simulink model "Model_PID"  (R2020b)
settings: Solver=ode4  StartTime=0.0  StopTime=1000  FixedStep=0.01  RelTol=1e-3
undefined symbols (not defined in the file): B, D, E_c, gama_c, gama_vjet, H, Iz, Kdpsi, Kdx, Kipsi, Kix, Kppsi, Kpx, Kurs_poc, L, m, N_c, Nr, Nrdot, Nrr, Nv, Polozaj_poc_E, Polozaj_poc_N, r_o, ro, ro_vj, T, V_c, V_vj, Xu, Xudot, Yr, Yrdot, Yv, Yvdot
libraries: simulink_extras x8, simulink x2
settings Model: Creator=Luka  LastModifiedBy=Luka
settings SolverCC: AlgebraicLoopSolver=LineSearch

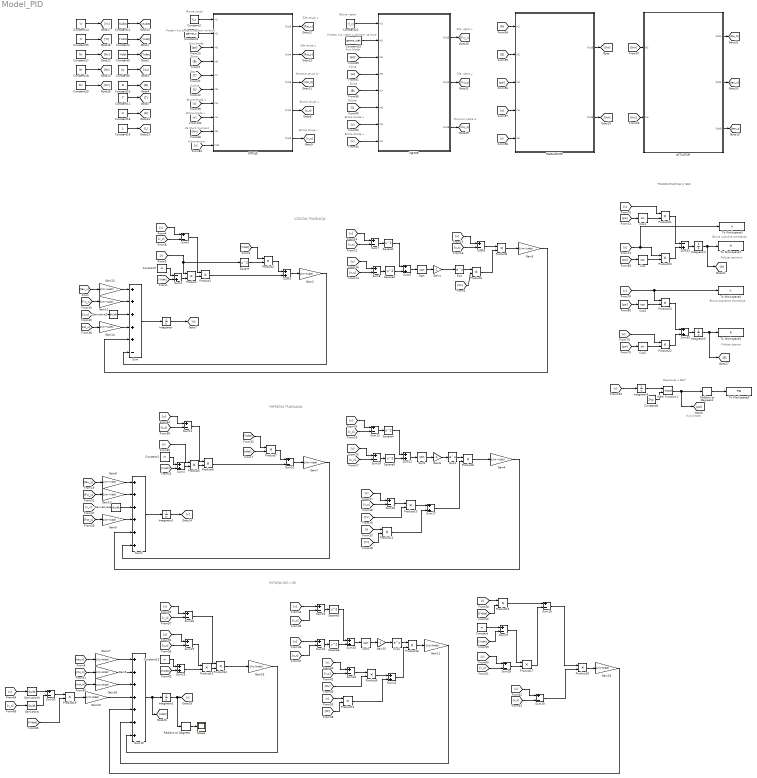
== system Model_PID ==
  note: Brzina struje v
  note: Brzina struje u
  note: Kutna brzina
  note: UZDUŽNA TRANSLACIJA
  note: POPREČNA TRANSLACIJA
  note: ROTACIJA OKO z OSI
  note: TRANSFORAMCIJA U NED
  note: Položaj istočno
  note: Položaj sjeverno
  note: Brzina uzdužna translacija
  note: Brzina poprečna translacija
  note: Visina
  note: Sila vjetra x
  note: Brzina vjetra
  note: Sila vjetra y
  note: Moment vjetra N
  note: Duljina
  note: Širina
  note: Pocetni kut vjetra s obzirom na brod
  note: Kurs broda
  note: Brzina broda u
  note: Brzina broda v
  note: Sila struje y
  note: Gaz
  note: Brzina struje
  note: Pocetni kut struje s obzirom na brod
  note: Sila struje x
  note: Duljina
  note: Kurs broda
  note: Moment struje N
  note: Širina
  note: Za Munk moment
  note: Brzina broda v
  note: Brzina broda u
  note: Mapiranje u 360°
  note: Kurs broda
  AKTUATOR : Subsystem
  Constant{,1,7,13} (4 alike) : Constant  Value=m
  Constant10 : Constant  Value=B
  Constant11 : Constant  Value=T
  Constant12 : Constant  Value=Xudot
  Constant14 : Constant  Value=Yv
  Constant15 : Constant  Value=Yr
  Constant16 : Constant  Value=H
  Constant17 : Constant  Value=Nv
  Constant18 : Constant  Value=Nr
  Constant19 : Constant  Value=L
  Constant2 : Constant  Value=V_c
  Constant20 : Constant  Value=Nrr
  Constant24 : Constant  Value=V_vj
  Constant25 : Constant  Value=gama_vjet
  Constant3 : Constant  Value=gama_c
  Constant4 : Constant  Value=Yvdot
  Constant5 : Constant  Value=Yrdot
  Constant6 : Constant  Value=Xu
  Constant8 : Constant  Value=2*pi
  Cos : Trigonometry  Operator=cos
  Cos1 : Trigonometry
  Cos2 : Trigonometry
  Cos3 : Trigonometry  Operator=cos
  Derivative{,1..3} (4 alike) : Derivative
  Exp : Math  SaturateOnIntegerOverflow=on
  Exp1 : Math  SaturateOnIntegerOverflow=on
  Exp2 : Math  SaturateOnIntegerOverflow=on
  Gain1 : Gain  Gain=-1
  Gain{4,7..10} (5 alike) : Gain  Gain=1/(m-Yvdot)
  Gain{5,11,16..20} (7 alike) : Gain  Gain=1/(Iz-Nrdot)
  Gain{2..3,12..14} (5 alike) : Gain  Gain=1/(m-Xudot)
  Gain15 : Gain  Gain=-1
  Gain6 : Gain  Gain=-1
  Integrator : Integrator
  Integrator1 : Integrator
  Integrator2 : Integrator
  Integrator4 : Integrator  InitialCondition=Polozaj_poc_N
  Integrator5 : Integrator  InitialCondition=Polozaj_poc_E
  Integrator6 : Integrator  InitialCondition=Kurs_poc
  Math Function1 : Math  Operator=mod  SaturateOnIntegerOverflow=on
  Product{,1..23} (24 alike) : Product
  REGULATOR : Subsystem
  Radians to Degrees : simulink_extras/Transformations/Radians to Degrees
  Radians to Degrees1 : simulink_extras/Transformations/Radians to Degrees
  STRUJE : Subsystem
  Scope : Scope
  Sqrt : Sqrt  SaturateOnIntegerOverflow=on
  Sqrt1 : Sqrt  SaturateOnIntegerOverflow=on
  Sqrt2 : Sqrt  SaturateOnIntegerOverflow=on
  Square{,1..6} (7 alike) : Math  Operator=square  SaturateOnIntegerOverflow=on
  Sum : Sum  Inputs=+++++-
  Sum1 : Sum  Inputs=++++++
  Sum{5,7..11,13..14,16,18..19,21..23,26..30} (19 alike) : Sum  Inputs=+-
  Sum{3..4,6,12,17,20,24..25,35} (9 alike) : Sum
  Sum15 : Sum  Inputs=+++++++
  Sum2 : Sum  Inputs=-+
  Sum32 : Sum  Inputs=-+
  To Workspace1 : ToWorkspace  VariableName=N  SaveFormat=Timeseries  SampleTime=-1
  To Workspace2 : ToWorkspace  VariableName=E  SaveFormat=Timeseries  SampleTime=-1
  To Workspace3 : ToWorkspace  VariableName=U  SaveFormat=Timeseries  SampleTime=-1
  To Workspace4 : ToWorkspace  VariableName=V  SaveFormat=Timeseries  SampleTime=-1
  To Workspace5 : ToWorkspace  VariableName=PSI  SaveFormat=Timeseries  SampleTime=-1
  VJETAR : Subsystem
  wires:
  Sum/1 -> Integrator/1
  Constant4/1 -> [Yvdot]
  Constant5/1 -> [Yrdot]
  Constant6/1 -> [Xu]
  Constant7/1 -> Sum2/1
  Sum2/1 -> Product/2
  [r] -> Square/1, Product/1
  [Yvdot] -> Sum2/2
  Constant10/1 -> [B]
  Constant11/1 -> [T]
  Product/1 -> Product1/2
  Product1/1 -> Sum3/2
  Square/1 -> Product2/2
  [Yrdot] -> Product2/1
  Product2/1 -> Sum3/1
  [v] -> Sum5/1
  [v_c] -> Sum5/2
  Sum5/1 -> Product1/1
  [v] -> Sum7/1
  [v_c] -> Sum7/2
  Sum7/1 -> Square1/1
  [u_c] -> Sum8/2
  [u] -> Sum8/1
  Sum8/1 -> Square2/1
  Square2/1 -> Sum6/2
  Square1/1 -> Sum6/1
  Sum6/1 -> Sqrt/1
  Exp/1 -> Product3/1
  [Xu] -> Product3/2
  [u_c] -> Sum9/2
  [u] -> Sum9/1
  Product3/1 -> Product4/2
  Gain2/1 -> Sum/6
  Derivative1/1 -> Sum1/3
  [Fst_y] -> Gain9/1
  Gain7/1 -> Sum1/6
  Gain6/1 -> Exp1/1
  Sqrt1/1 -> Gain6/1
  [u] -> Sum11/1
  Product6/1 -> Sum10/2
  [v] -> Sum13/1
  Gain10/1 -> Sum1/2
  [u_c] -> Sum11/2
  Square5/1 -> Sum12/2
  Sum10/1 -> Gain7/1
  Product5/1 -> Product6/2
  [v_c] -> Derivative1/1
  [u_c] -> Sum14/2
  Sum13/1 -> Square4/1
  [u] -> Sum14/1
  Exp1/1 -> Product8/1
  [r] -> Product5/1
  Sum12/1 -> Sqrt1/1
  Sum14/1 -> Square5/1
  [Yrdot] -> Product7/1
  Sum1/1 -> Integrator1/1
  [v_c] -> Sum13/2
  [Fvj_y] -> Gain10/1
  Sum11/1 -> Product6/1
  Product7/1 -> Sum10/1
  Gain8/1 -> Sum1/1
  Integrator1/1 -> [v]
  Square4/1 -> Sum12/1
  [Xudot] -> Sum4/2
  Constant1/1 -> Sum4/1
  Sum4/1 -> Product5/2
  Product8/1 -> Gain4/1
  Product4/1 -> Gain3/1
  Derivative2/1 -> Sum/3
  [Fst_x] -> Gain14/1
  Gain12/1 -> Sum/2
  [Fvj_x] -> Gain12/1
  [tau_x] -> Gain13/1
  [u_c] -> Derivative2/1
  Sum3/1 -> Gain2/1
  Constant12/1 -> [Xudot]
  [rdot] -> Product7/2
  [v] -> Sum16/1
  [v_c] -> Sum16/2
  [Yv] -> Product10/2
  Product10/1 -> Sum17/1
  [r] -> Product11/1
  [Yr] -> Product11/2
  Product11/1 -> Sum17/2
  Sum17/1 -> Product8/2
  Constant14/1 -> [Yv]
  Constant15/1 -> [Yr]
  [v_c] -> Sum23/2
  Gain16/1 -> Sum15/7
  Gain18/1 -> Sum15/3
  [Mvj_N] -> Gain5/1
  Product14/1 -> Gain16/1
  Gain11/1 -> Sum15/6
  Product16/1 -> Gain11/1
  Gain15/1 -> Exp2/1
  Product12/1 -> Sum24/2
  [u] -> Sum19/1
  Sqrt2/1 -> Gain15/1
  Sum24/1 -> Product16/2
  [r] -> Product12/1
  Square6/1 -> Sum20/2
  [u_c] -> Sum19/2
  Gain5/1 -> Sum15/2
  [Nr] -> Product12/2
  Sum25/1 -> Product13/2
  [Xudot] -> Sum25/2
  Constant13/1 -> Sum25/1
  Gain17/1 -> Sum15/1
  [v_c] -> Sum21/2
  Square3/1 -> Sum20/1
  Sum23/1 -> Product9/1
  [Nv] -> Product9/2
  Sum19/1 -> Product13/1
  [v] -> Sum21/1
  Sum22/1 -> Square6/1
  Product9/1 -> Sum24/1
  Sum20/1 -> Sqrt2/1
  Sum15/1 -> Integrator2/1, [rdot]
  Sum21/1 -> Square3/1
  Exp2/1 -> Product16/1
  [u_c] -> Sum22/2
  [Mst_N] -> Gain18/1
  Product13/1 -> Product14/2
  [u] -> Sum22/1
  [v] -> Sum23/1
  [v_c] -> Sum26/2
  [v] -> Sum26/1
  Sum26/1 -> Product14/1
  Constant17/1 -> [Nv]
  Constant18/1 -> [Nr]
  [r] -> Product15/1
  [Yrdot] -> Product15/2
  Product15/1 -> Sum18/1
  Constant/1 -> Sum27/1
  [Yvdot] -> Sum27/2
  [v_c] -> Sum28/2
  [v] -> Sum28/1
  Sum28/1 -> Product17/2
  Sum27/1 -> Product17/1
  Product17/1 -> Sum18/2
  Sum29/1 -> Product18/2
  [u_c] -> Sum29/2
  [u] -> Sum29/1
  Sum18/1 -> Product18/1
  Product18/1 -> Gain19/1
  Gain19/1 -> Sum15/5
  [v_c] -> Derivative/1
  Derivative/1 -> Sum30/2
  [Yrdot] -> Product19/2
  Sum30/1 -> Product19/1
  Product19/1 -> Gain20/1
  Gain20/1 -> Sum15/4
  Product20/1 -> Sum32/2
  [psi] -> Cos/1
  Cos/1 -> Product20/2
  [u] -> To Workspace3/1, Product20/1
  Cos1/1 -> Product21/2
  [psi] -> Cos1/1
  [v] -> Product21/1
  Product21/1 -> Sum32/1
  Sum32/1 -> Integrator4/1
  Integrator4/1 -> [N], To Workspace1/1
  Cos3/1 -> Product23/2
  Product22/1 -> Sum35/2
  [u] -> Product22/1
  Product23/1 -> Sum35/1
  [psi] -> Cos2/1
  Sum35/1 -> Integrator5/1
  Cos2/1 -> Product22/2
  [psi] -> Cos3/1
  [v] -> To Workspace4/1, Product23/1
  Constant16/1 -> [H]
  Constant19/1 -> [L]
  Constant20/1 -> [Nrr]
  Integrator5/1 -> [E], To Workspace2/1
  [tau_y] -> Gain8/1
  [tau_N] -> Gain17/1
  [B] -> VJETAR/5(In7)
  VJETAR/1(Out3) -> [Fvj_x]
  [L] -> VJETAR/6(In8)
  Constant24/1 -> VJETAR/1(In1)
  VJETAR/3(Out5) -> [Mvj_N]
  [psi] -> VJETAR/3(In5)
  [H] -> VJETAR/4(In6)
  Constant25/1 -> VJETAR/2(In2)
  VJETAR/2(Out4) -> [Fvj_y]
  [u] -> VJETAR/7(In3)
  [v] -> VJETAR/8(In4)
  [r] -> REGULATOR/5(In5)
  [u] -> REGULATOR/4(In4)
  [N] -> REGULATOR/1(In1)
  [psi] -> REGULATOR/3(In3)
  [E] -> REGULATOR/2(In2)
  Constant2/1 -> STRUJE/1(In1)
  [B] -> STRUJE/4(In6)
  [psi] -> STRUJE/3(In5)
  [L] -> STRUJE/6(In8)
  [T] -> STRUJE/5(In7)
  STRUJE/2(Out4) -> [Fst_y]
  STRUJE/3(Out5) -> [Mst_N]
  Constant3/1 -> STRUJE/2(In2)
  [v] -> STRUJE/8(In4)
  [u] -> STRUJE/7(In3)
  [Nrr] -> STRUJE/9(In9)
  [r] -> STRUJE/10(In10)
  Radians to Degrees1/1 -> To Workspace5/1
  Math Function1/1 -> [psi], Radians to Degrees1/1
  Constant8/1 -> Math Function1/2
  Integrator6/1 -> Math Function1/1
  [r] -> Integrator6/1
  STRUJE/4(Out1) -> [u_c]
  STRUJE/5(Out2) -> [v_c]
  [v] -> Derivative3/1
  Derivative3/1 -> Sum30/1
  STRUJE/1(Out3) -> [Fst_x]
  Sqrt/1 -> Gain1/1
  Gain1/1 -> Exp/1
  Sum9/1 -> Product4/1
  Gain3/1 -> Sum/5
  Sum16/1 -> Product10/1
  Gain4/1 -> Sum1/5
  Gain9/1 -> Sum1/4
  Gain14/1 -> Sum/4
  Integrator/1 -> [u]
  Gain13/1 -> Sum/1
  REGULATOR/1(Out3) -> [Urx]
  REGULATOR/2(Out5) -> [Urn]
  AKTUATOR/2(Out2) -> [tau_x]
  AKTUATOR/1(Out1) -> [tau_N]
  AKTUATOR/3(Out6) -> [tau_y]
  [Urx] -> AKTUATOR/2(In4)
  [Urn] -> AKTUATOR/1(In2)
  Integrator2/1 -> Radians to Degrees/1, [r]
  Radians to Degrees/1 -> Scope/1

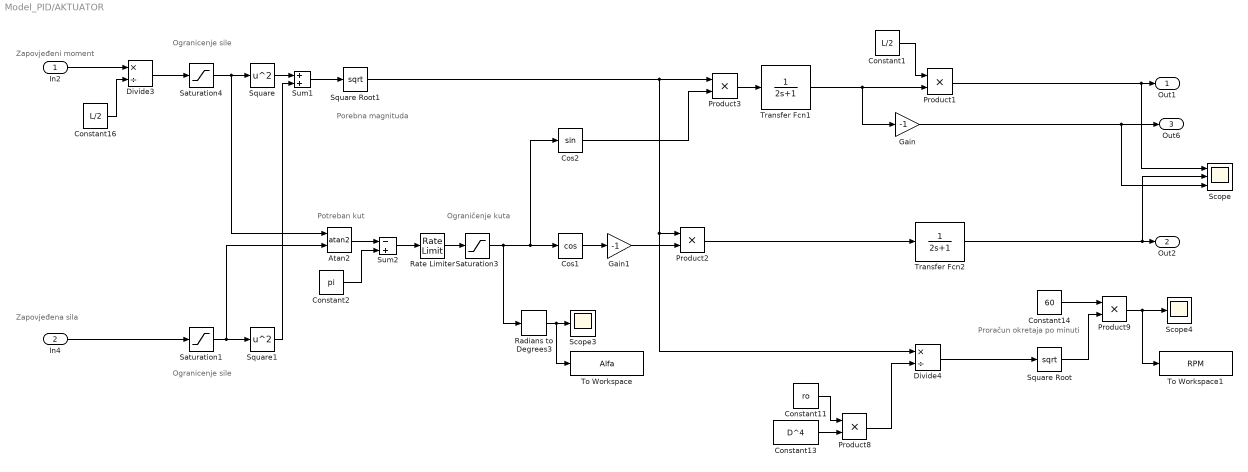
== system Model_PID/AKTUATOR ==
  note: Porebna magnituda
  note: Zapovjeđeni moment
  note: Zapovjeđena sila
  note: Proračun okretaja po minuti
  note: Ograničenje kuta
  note: Ogranicenje sile
  note: Potreban kut
  note: Ogranicenje sile
  In2 : Inport
  In4 : Inport  Port=2
  Atan2 : Trigonometry  Operator=atan2
  Constant1 : Constant  Value=L/2
  Constant11 : Constant  Value=ro
  Constant13 : Constant  Value=D^4
  Constant14 : Constant  Value=60
  Constant16 : Constant  Value=L/2
  Constant2 : Constant  Value=pi
  Cos1 : Trigonometry  Operator=cos
  Cos2 : Trigonometry
  Divide3 : Product  Inputs=*/
  Divide4 : Product  Inputs=*/
  Gain : Gain  Gain=-1
  Gain1 : Gain  Gain=-1
  Product{1..3,8..9} (5 alike) : Product
  Radians to Degrees3 : simulink_extras/Transformations/Radians to Degrees
  Rate Limiter : RateLimiter  RisingSlewLimit=40*pi/180  FallingSlewLimit=-40*pi/180  SampleTimeMode=inherited
  Saturation1 : Saturate  UpperLimit=300  LowerLimit=0
  Saturation3 : Saturate  UpperLimit=250*pi/180  LowerLimit=110*pi/180
  Saturation4 : Saturate  UpperLimit=280  LowerLimit=-280
  Scope : Scope  NumInputPorts=3
  Scope3 : Scope
  Scope4 : Scope
  Square : Math  Operator=square  SaturateOnIntegerOverflow=on
  Square Root : Sqrt  SaturateOnIntegerOverflow=on
  Square Root1 : Sqrt  SaturateOnIntegerOverflow=on
  Square1 : Math  Operator=square  SaturateOnIntegerOverflow=on
  Sum1 : Sum
  Sum2 : Sum  Inputs=-+
  To Workspace : ToWorkspace  VariableName=Alfa  SaveFormat=Timeseries  SampleTime=-1
  To Workspace1 : ToWorkspace  VariableName=RPM  SaveFormat=Timeseries  SampleTime=-1
  Transfer Fcn1 : TransferFcn  Denominator=[2 1]
  Transfer Fcn2 : TransferFcn  Denominator=[2 1]
  Out1 : Outport
  Out2 : Outport  Port=2
  Out6 : Outport  Port=3
  wires:
  Sum2/1 -> Rate Limiter/1
  Product8/1 -> Divide4/2
  Gain/1 -> Scope/3, Out6/1
  Sum1/1 -> Square Root1/1
  Constant16/1 -> Divide3/2
  Saturation3/1 -> Cos2/1, Cos1/1, Radians to Degrees3/1
  Saturation4/1 -> Atan2/1, Square/1
  Divide3/1 -> Saturation4/1
  Cos1/1 -> Gain1/1
  Gain1/1 -> Product2/2
  In4/1 -> Saturation1/1
  Constant11/1 -> Product8/1
  Rate Limiter/1 -> Saturation3/1
  Transfer Fcn1/1 -> Gain/1, Product1/2
  Square1/1 -> Sum1/2
  Square/1 -> Sum1/1
  Product3/1 -> Transfer Fcn1/1
  Cos2/1 -> Product3/2
  Atan2/1 -> Sum2/1
  In2/1 -> Divide3/1
  Product2/1 -> Transfer Fcn2/1
  Product9/1 -> To Workspace1/1, Scope4/1
  Product1/1 -> Scope/1, Out1/1
  Square Root/1 -> Product9/2
  Transfer Fcn2/1 -> Scope/2, Out2/1
  Constant13/1 -> Product8/2
  Divide4/1 -> Square Root/1
  Square Root1/1 -> Divide4/1, Product2/1, Product3/1
  Saturation1/1 -> Atan2/2, Square1/1
  Radians to Degrees3/1 -> Scope3/1, To Workspace/1
  Constant2/1 -> Sum2/2
  Constant1/1 -> Product1/1
  Constant14/1 -> Product9/1

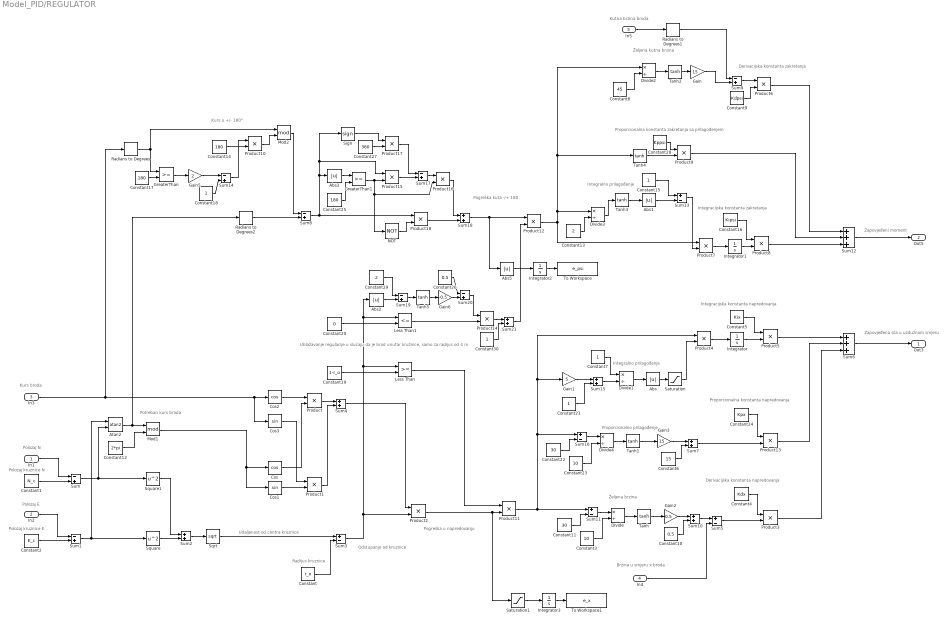
== system Model_PID/REGULATOR ==
  note: Kurs u +/- 180°
  note: Proporcionalno prilagođenje
  note: Udaljenost od centra kruznice
  note: Ublažavanje regulacije u slučaju da je brod unutar kružnice, samo za radijus od 4 m
  note: Pogreška u napredovanju
  note: Radijus kruznice
  note: Željena kutna brzina
  note: Proporcionalna konstanta napredovanja
  note: Pogreška kuta -/+ 180
  note: Zapovjeđena sila u uzdužnom smjeru
  note: Zapovjeđeni moment
  note: Kutna brzina broda
  note: Integralno prilagođenje
  note: Derivacijska konstanta napredovanja
  note: Željena brzina
  note: Brzina u smjeru x broda
  note: Kurs broda
  note: Odstupanje od kruznice
  note: Potreban kurs broda
  note: Polozaj N
  note: Polozaj E
  note: Polozaj kruznice N
  note: Polozaj kruznice E
  note: Integracijska konstanta napredovanja
  note: Derivacijska konstanta zakretanja
  note: Integralno prilagođenje
  note: Integracijska konstanta zakretanja
  note: Proporcionalna konstanta zakretanja sa prilagođenjem
  In1 : Inport
  In2 : Inport  Port=2
  In3 : Inport  Port=3
  In4 : Inport  Port=4
  In5 : Inport  Port=5
  Abs{,1..3,5} (5 alike) : Abs
  Atan2 : Trigonometry  Operator=atan2
  Constant : Constant  Value=r_o
  Constant1 : Constant  Value=N_c
  Constant10 : Constant  Value=0.5
  Constant11 : Constant  Value=30
  Constant12 : Constant  Value=2*pi
  Constant13 : Constant  Value=2
  Constant14 : Constant  Value=180
  Constant{7,15,18,21,30} (5 alike) : Constant
  Constant16 : Constant  Value=Kipsi
  Constant17 : Constant  Value=180
  Constant19 : Constant  Value=1-r_o
  Constant2 : Constant  Value=E_c
  Constant20 : Constant  Value=0
  Constant22 : Constant  Value=30
  Constant23 : Constant  Value=10
  Constant24 : Constant  Value=Kpx
  Constant25 : Constant  Value=180
  Constant26 : Constant  Value=0.5
  Constant27 : Constant  Value=360
  Constant28 : Constant  Value=Kppsi
  Constant29 : Constant  Value=2
  Constant3 : Constant  Value=10
  Constant4 : Constant  Value=Kdx
  Constant5 : Constant  Value=Kix
  Constant6 : Constant  Value=15
  Constant8 : Constant  Value=45
  Constant9 : Constant  Value=Kdpsi
  Cos : Trigonometry  Operator=cos
  Cos1 : Trigonometry
  Cos2 : Trigonometry  Operator=cos
  Cos3 : Trigonometry
  Divide{,1..4} (5 alike) : Product  Inputs=*/
  Gain : Gain  Gain=15
  Gain1 : Gain  Gain=5
  Gain2 : Gain  Gain=0.5
  Gain3 : Gain  Gain=15
  Gain5 : Gain  Gain=2
  Gain6 : Gain  Gain=-0.5
  GreaterThan : RelationalOperator  OutDataTypeStr=boolean  RndMeth=Simplest
  GreaterThan1 : RelationalOperator  OutDataTypeStr=boolean  RndMeth=Simplest
  Integrator{,1..3} (4 alike) : Integrator
  Less Than : RelationalOperator  OutDataTypeStr=boolean  RndMeth=Simplest
  Less Than1 : RelationalOperator  Operator=<=  OutDataTypeStr=boolean  RndMeth=Simplest
  Mod1 : Math  Operator=mod  SaturateOnIntegerOverflow=on
  Mod2 : Math  Operator=mod  SaturateOnIntegerOverflow=on
  NOT : Logic  Operator=NOT  IconShape=distinctive  AllPortsSameDT=off  OutDataTypeStr=boolean
  Product{,1..18} (19 alike) : Product
  Radians to Degrees : simulink_extras/Transformations/Radians to Degrees
  Radians to Degrees1 : simulink_extras/Transformations/Radians to Degrees
  Radians to Degrees2 : simulink_extras/Transformations/Radians to Degrees
  Saturation : Saturate  UpperLimit=1  LowerLimit=0
  Saturation1 : Saturate  UpperLimit=50  LowerLimit=0
  Sign : Signum
  Sqrt : Sqrt  SaturateOnIntegerOverflow=on
  Square : Math  Operator=square  SaturateOnIntegerOverflow=on
  Square1 : Math  Operator=square  SaturateOnIntegerOverflow=on
  Sum{,1,8..9,14,17,19..20} (8 alike) : Sum  Inputs=-+
  Sum{2,4,7,10,15,18,21} (7 alike) : Sum
  Sum{3,5,11,13,16} (5 alike) : Sum  Inputs=+-
  Sum12 : Sum  Inputs=+++
  Sum6 : Sum  Inputs=+++
  Tanh{,1..5} (6 alike) : Trigonometry  Operator=tanh
  To Workspace : ToWorkspace  VariableName=e_psi  SaveFormat=Timeseries  SampleTime=-1
      settings: Decimation=2
  To Workspace1 : ToWorkspace  VariableName=e_x  SaveFormat=Timeseries  SampleTime=-1
      settings: Decimation=2
  Out3 : Outport
  Out5 : Outport  Port=2
  wires:
  Constant1/1 -> Sum/2
  In1/1 -> Sum/1
  Constant2/1 -> Sum1/2
  In2/1 -> Sum1/1
  Sum1/1 -> Square/1, Atan2/1
  Sum/1 -> Square1/1, Atan2/2
  Square1/1 -> Sum2/1
  Square/1 -> Sum2/2
  Sum2/1 -> Sqrt/1
  Sqrt/1 -> Sum3/1
  Constant/1 -> Sum3/2
  Atan2/1 -> Radians to Degrees2/1, Mod1/1
  In3/1 -> Cos3/1, Cos2/1, Radians to Degrees/1
  Cos2/1 -> Product/1
  Cos/1 -> Product/2
  Product/1 -> Sum4/1
  Cos1/1 -> Product1/2
  Cos3/1 -> Product1/1
  Product1/1 -> Sum4/2
  Sum4/1 -> Product2/1
  Constant3/1 -> Divide/2
  Divide/1 -> Tanh/1
  Constant4/1 -> Product3/1
  Divide1/1 -> Abs/1
  Constant7/1 -> Divide1/1
  Abs/1 -> Saturation/1
  Product4/1 -> Integrator/1
  Integrator/1 -> Product5/2
  Constant5/1 -> Product5/1
  Constant8/1 -> Divide2/2
  Divide2/1 -> Tanh2/1
  Tanh2/1 -> Gain/1
  In5/1 -> Radians to Degrees1/1
  Sum9/1 -> Product6/1
  Constant9/1 -> Product6/2
  Constant12/1 -> Mod1/2
  Radians to Degrees2/1 -> Sum8/2
  Mod1/1 -> Cos1/1, Cos/1
  Constant10/1 -> Sum10/2
  Sum10/1 -> Sum5/1
  Constant11/1 -> Sum11/2
  Sum11/1 -> Divide/1
  Sum12/1 -> Out5/1
  Divide3/1 -> Tanh3/1
  Tanh3/1 -> Abs1/1
  Constant13/1 -> Divide3/2
  Constant15/1 -> Sum13/1
  Integrator1/1 -> Product8/2
  Product7/1 -> Integrator1/1
  Constant16/1 -> Product8/1
  Sum13/1 -> Product7/2
  Constant18/1 -> Sum14/2
  Constant19/1 -> Less Than/2
  Constant20/1 -> Less Than1/2
  Sum3/1 -> Product2/2, Less Than/1, Abs2/1, Less Than1/1
  In4/1 -> Sum5/2
  Sum5/1 -> Product3/2
  Gain1/1 -> Sum15/1
  Sum15/1 -> Divide1/2
  Constant21/1 -> Sum15/2
  Constant22/1 -> Sum16/2
  Divide4/1 -> Tanh1/1
  Constant23/1 -> Divide4/2
  Constant6/1 -> Sum7/2
  Sum16/1 -> Divide4/1
  Tanh1/1 -> Gain3/1
  Gain3/1 -> Sum7/1
  Sum7/1 -> Product13/2
  Constant24/1 -> Product13/1
  Tanh/1 -> Gain2/1
  Gain2/1 -> Sum10/1
  Radians to Degrees1/1 -> Sum9/1
  Product11/1 -> Sum16/1, Gain1/1, Product4/1, Sum11/1
  Saturation/1 -> Product4/2
  Gain5/1 -> Sum14/1
  Radians to Degrees/1 -> GreaterThan/1, Mod2/1
  Constant17/1 -> GreaterThan/2
  GreaterThan/1 -> Gain5/1
  Sum14/1 -> Product10/1
  Mod2/1 -> Sum8/1
  Constant14/1 -> Product10/2
  Product10/1 -> Mod2/2
  Abs3/1 -> GreaterThan1/1
  Constant25/1 -> GreaterThan1/2
  GreaterThan1/1 -> NOT/1, Product16/2, Product15/2
  Sum8/1 -> Product15/1, Sign/1, Abs3/1, Product18/1
  Product15/1 -> Sum17/2
  Sum17/1 -> Product16/1
  Product16/1 -> Sum18/1
  Constant27/1 -> Product17/2
  Product17/1 -> Sum17/1
  Sum18/1 -> Product12/1, Abs5/1
  NOT/1 -> Product18/2
  Product18/1 -> Sum18/2
  Abs1/1 -> Sum13/2
  Sign/1 -> Product17/1
  Product6/1 -> Sum12/1
  Product12/1 -> Divide2/1, Tanh4/1, Divide3/1, Product7/1
  Tanh4/1 -> Product9/2
  Constant28/1 -> Product9/1
  Product9/1 -> Sum12/2
  Abs2/1 -> Sum19/2
  Constant29/1 -> Sum19/1
  Sum19/1 -> Tanh5/1
  Tanh5/1 -> Gain6/1
  Gain6/1 -> Sum20/2
  Constant26/1 -> Sum20/1
  Sum20/1 -> Product14/1
  Less Than1/1 -> Product14/2
  Product14/1 -> Sum21/1
  Constant30/1 -> Sum21/2
  Product8/1 -> Sum12/3
  Gain/1 -> Sum9/2
  Product5/1 -> Sum6/1
  Product13/1 -> Sum6/2
  Product3/1 -> Sum6/3
  Sum6/1 -> Out3/1
  Integrator2/1 -> To Workspace/1
  Product2/1 -> Saturation1/1, Product11/2
  Integrator3/1 -> To Workspace1/1
  Saturation1/1 -> Integrator3/1
  Abs5/1 -> Integrator2/1
  Sum21/1 -> Product12/2
  Less Than/1 -> Product11/1

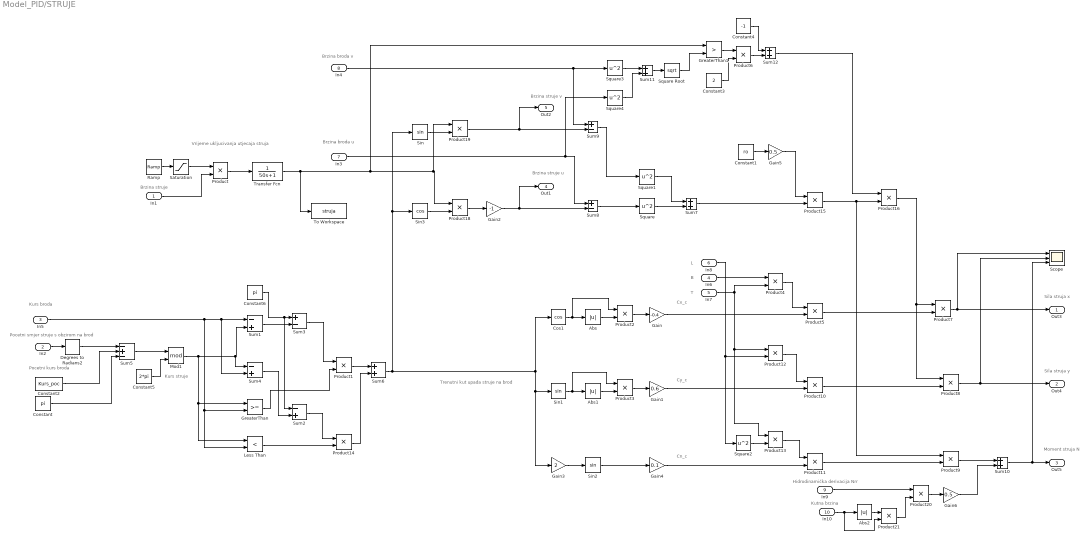
== system Model_PID/STRUJE ==
  note: Brzina struje v
  note: Kutna brzina
  note: Hidrodinamička derivacija Nrr
  note: Brzina broda u
  note: Brzina broda v
  note: Trenutni kut upada struje na brod
  note: Vrijeme ukljucivanja utjecaja struja
  note: Sila struja x
  note: B
  note: Cx_c
  note: Kurs broda
  note: Pocetni smjer struje s obzirom na brod
  note: Brzina struje
  note: Kurs struje
  note: Cy_c
  note: Cn_c
  note: T
  note: Sila struja y
  note: Moment struja N
  note: L
  note: Pocetni kurs broda
  note: Brzina struje u
  In1 : Inport
  In2 : Inport  Port=2
  In5 : Inport  Port=3
  In6 : Inport  Port=4
  In7 : Inport  Port=5
  In8 : Inport  Port=6
  In3 : Inport  Port=7
  In4 : Inport  Port=8
  In9 : Inport  Port=9
  In10 : Inport  Port=10
  Abs : Abs
  Abs1 : Abs
  Abs2 : Abs
  Constant : Constant  Value=pi
  Constant1 : Constant  Value=ro
  Constant2 : Constant  Value=Kurs_poc
  Constant3 : Constant  Value=2
  Constant4 : Constant  Value=-1
  Constant5 : Constant  Value=2*pi
  Constant6 : Constant  Value=pi
  Cos1 : Trigonometry  Operator=cos
  Degrees to Radians2 : simulink_extras/Transformations/Degrees to Radians
  Gain : Gain  Gain=-0.4
  Gain1 : Gain  Gain=0.6
  Gain2 : Gain  Gain=-1
  Gain3 : Gain  Gain=2
  Gain4 : Gain  Gain=0.1
  Gain5 : Gain  Gain=0.5
  Gain6 : Gain  Gain=0.5
  GreaterThan : RelationalOperator  OutDataTypeStr=boolean  RndMeth=Simplest
  GreaterThan1 : RelationalOperator  Operator=>  OutDataTypeStr=boolean  RndMeth=Simplest
  Less Than : RelationalOperator  Operator=<  OutDataTypeStr=boolean  RndMeth=Simplest
  Mod1 : Math  Operator=mod  SaturateOnIntegerOverflow=on
  Product{,1..16,18..21} (21 alike) : Product
  Ramp : simulink/Sources/Ramp  slope=0.002  start=0  InitialOutput=0
  Saturation : Saturate  UpperLimit=1  LowerLimit=-1
  Scope : Scope  NumInputPorts=3
  Sin : Trigonometry
  Sin1 : Trigonometry
  Sin2 : Trigonometry
  Sin3 : Trigonometry  Operator=cos
  Square{,1..4} (5 alike) : Math  Operator=square  SaturateOnIntegerOverflow=on
  Square Root : Sqrt  SaturateOnIntegerOverflow=on
  Sum1 : Sum  Inputs=-+
  Sum{6..7,10..12} (5 alike) : Sum
  Sum2 : Sum  Inputs=-+
  Sum3 : Sum  Inputs=+-
  Sum4 : Sum  Inputs=-+
  Sum5 : Sum  Inputs=-+-
  Sum8 : Sum  Inputs=+-
  Sum9 : Sum  Inputs=+-
  To Workspace : ToWorkspace  VariableName=struja  SaveFormat=Timeseries  SampleTime=-1
  Transfer Fcn : TransferFcn  Denominator=[50 1]
  Out3 : Outport
  Out4 : Outport  Port=2
  Out5 : Outport  Port=3
  Out1 : Outport  Port=4
  Out2 : Outport  Port=5
  wires:
  Cos1/1 -> Product2/1, Abs/1
  Abs/1 -> Product2/2
  Product2/1 -> Gain/1
  Sin1/1 -> Product3/1, Abs1/1
  Abs1/1 -> Product3/2
  Product3/1 -> Gain1/1
  Gain3/1 -> Sin2/1
  Sin2/1 -> Gain4/1
  Constant1/1 -> Gain5/1
  In6/1 -> Product4/1
  In7/1 -> Product12/1, Product13/1, Product4/2
  Product4/1 -> Product5/1
  Gain/1 -> Product5/2
  In8/1 -> Product12/2, Square2/1
  Gain1/1 -> Product10/2
  Gain4/1 -> Product11/2
  Product12/1 -> Product10/1
  Square2/1 -> Product13/2
  Product13/1 -> Product11/1
  Sum5/1 -> Mod1/1
  In2/1 -> Degrees to Radians2/1
  Degrees to Radians2/1 -> Sum5/1
  Constant/1 -> Sum5/3
  Constant5/1 -> Mod1/2
  Mod1/1 -> Sum4/1, Sum1/2, Less Than/1, GreaterThan/1
  In5/1 -> Less Than/2, GreaterThan/2, Sum4/2, Sum1/1
  Constant6/1 -> Sum2/1, Sum3/1
  Sum1/1 -> Sum3/2
  GreaterThan/1 -> Product1/2
  Sum3/1 -> Product1/1
  Less Than/1 -> Product14/2
  Sum4/1 -> Sum2/2
  Sum2/1 -> Product14/1
  Product1/1 -> Sum6/1
  Sum6/1 -> Gain3/1, Sin1/1, Cos1/1, Sin3/1, Sin/1
  Product14/1 -> Sum6/2
  Ramp/1 -> Saturation/1
  Saturation/1 -> Product/1
  Sin3/1 -> Product18/2
  Square/1 -> Sum7/2
  Gain5/1 -> Product15/1
  Square1/1 -> Sum7/1
  Sin/1 -> Product19/2
  Product21/1 -> Product20/2
  In9/1 -> Product20/1
  Abs2/1 -> Product21/1
  In10/1 -> Product21/2, Abs2/1
  Product19/1 -> Sum9/2, Out2/1
  Product18/1 -> Gain2/1
  Sum8/1 -> Square/1
  Gain2/1 -> Sum8/2, Out1/1
  Product7/1 -> Out3/1, Scope/1
  Constant2/1 -> Sum5/2
  Product5/1 -> Product7/2
  Product10/1 -> Product8/2
  Product11/1 -> Product9/2
  Sum9/1 -> Square1/1
  Product8/1 -> Out4/1, Scope/2
  Sum10/1 -> Scope/3, Out5/1
  In4/1 -> Sum9/1, Square3/1
  Product/1 -> Transfer Fcn/1
  Transfer Fcn/1 -> To Workspace/1, GreaterThan1/1, Product19/1, Product18/1
  Product20/1 -> Gain6/1
  In1/1 -> Product/2
  In3/1 -> Square4/1, Sum8/1
  Square3/1 -> Sum11/1
  Square4/1 -> Sum11/2
  Sum11/1 -> Square Root/1
  Square Root/1 -> GreaterThan1/2
  GreaterThan1/1 -> Product6/1
  Constant3/1 -> Product6/2
  Product6/1 -> Sum12/2
  Constant4/1 -> Sum12/1
  Sum12/1 -> Product16/1
  Product9/1 -> Sum10/1
  Gain6/1 -> Sum10/2
  Product15/1 -> Product9/1, Product16/2
  Sum7/1 -> Product15/2
  Product16/1 -> Product8/1, Product7/1

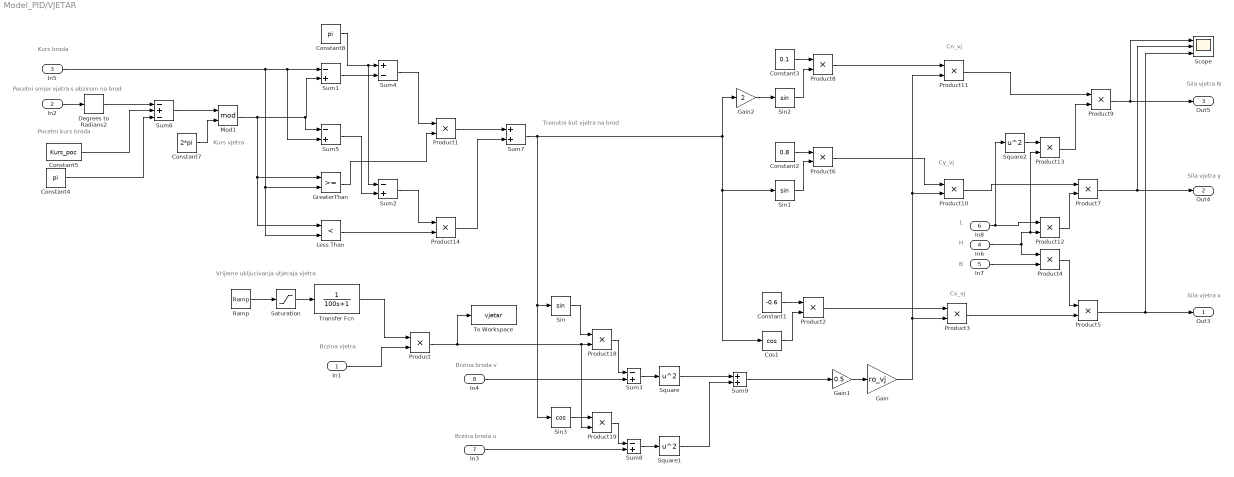
== system Model_PID/VJETAR ==
  note: Trenutni kut vjetra na brod
  note: Brzina broda v
  note: Brzina broda u
  note: Sila vjetra x
  note: H
  note: B
  note: Cx_vj
  note: Brzina vjetra
  note: Cy_vj
  note: Cn_vj
  note: Sila vjetra y
  note: Sila vjetra N
  note: L
  note: Pocetni kurs broda
  note: Kurs broda
  note: Pocetni smjer vjetra s obzirom na brod
  note: Kurs vjetra
  note: Vrijeme ukljucivanja utjecaja vjetra
  In1 : Inport
  In2 : Inport  Port=2
  In5 : Inport  Port=3
  In6 : Inport  Port=4
  In7 : Inport  Port=5
  In8 : Inport  Port=6
  In3 : Inport  Port=7
  In4 : Inport  Port=8
  Constant1 : Constant  Value=-0.6
  Constant2 : Constant  Value=0.8
  Constant3 : Constant  Value=0.1
  Constant4 : Constant  Value=pi
  Constant5 : Constant  Value=Kurs_poc
  Constant7 : Constant  Value=2*pi
  Constant8 : Constant  Value=pi
  Cos1 : Trigonometry  Operator=cos
  Degrees to Radians2 : simulink_extras/Transformations/Degrees to Radians
  Gain : Gain  Gain=ro_vj
  Gain1 : Gain  Gain=0.5
  Gain2 : Gain  Gain=2
  GreaterThan : RelationalOperator  OutDataTypeStr=boolean  RndMeth=Simplest
  Less Than : RelationalOperator  Operator=<  OutDataTypeStr=boolean  RndMeth=Simplest
  Mod1 : Math  Operator=mod  SaturateOnIntegerOverflow=on
  Product{,1..14,18..19} (17 alike) : Product
  Ramp : simulink/Sources/Ramp  slope=0.002  start=100  InitialOutput=0
  Saturation : Saturate  UpperLimit=1  LowerLimit=0
  Scope : Scope  NumInputPorts=3
  Sin : Trigonometry
  Sin1 : Trigonometry
  Sin2 : Trigonometry
  Sin3 : Trigonometry  Operator=cos
  Square : Math  Operator=square  SaturateOnIntegerOverflow=on
  Square1 : Math  Operator=square  SaturateOnIntegerOverflow=on
  Square2 : Math  Operator=square  SaturateOnIntegerOverflow=on
  Sum{1..3,5,8} (5 alike) : Sum  Inputs=-+
  Sum4 : Sum  Inputs=+-
  Sum6 : Sum  Inputs=-+-
  Sum7 : Sum
  Sum9 : Sum
  To Workspace : ToWorkspace  VariableName=vjetar  SaveFormat=Timeseries  SampleTime=-1
  Transfer Fcn : TransferFcn  Denominator=[100 1]
  Out3 : Outport
  Out4 : Outport  Port=2
  Out5 : Outport  Port=3
  wires:
  Gain1/1 -> Gain/1
  Constant1/1 -> Product2/1
  Cos1/1 -> Product2/2
  Product2/1 -> Product3/1
  Gain/1 -> Product10/2, Product11/2, Product3/2
  In6/1 -> Product4/1, Product13/2, Product12/2
  In7/1 -> Product4/2
  Product3/1 -> Product5/2
  Sin1/1 -> Product6/2
  Product6/1 -> Product10/1
  Constant2/1 -> Product6/1
  Constant3/1 -> Product8/1
  Sin2/1 -> Product8/2
  Product8/1 -> Product11/1
  Product11/1 -> Product9/1
  Product10/1 -> Product7/1
  Product4/1 -> Product5/1
  In8/1 -> Product12/1, Square2/1
  Product12/1 -> Product7/2
  Square2/1 -> Product13/1
  Product13/1 -> Product9/2
  Gain2/1 -> Sin2/1
  Sum1/1 -> Sum4/2
  Sum2/1 -> Product14/1
  Product1/1 -> Sum7/1
  Mod1/1 -> Sum5/1, Sum1/2, Less Than/1, GreaterThan/1
  Sum5/1 -> Sum2/2
  Constant7/1 -> Mod1/2
  Less Than/1 -> Product14/2
  Constant8/1 -> Sum2/1, Sum4/1
  Degrees to Radians2/1 -> Sum6/1
  In2/1 -> Degrees to Radians2/1
  GreaterThan/1 -> Product1/2
  Sum6/1 -> Mod1/1
  Constant5/1 -> Sum6/2
  In5/1 -> Less Than/2, GreaterThan/2, Sum5/2, Sum1/1
  Constant4/1 -> Sum6/3
  Product14/1 -> Sum7/2
  Sum4/1 -> Product1/1
  Sum7/1 -> Cos1/1, Sin1/1, Gain2/1, Sin3/1, Sin/1
  Ramp/1 -> Saturation/1
  Product9/1 -> Out5/1, Scope/1
  Product5/1 -> Out3/1, Scope/3
  Saturation/1 -> Transfer Fcn/1
  Product7/1 -> Out4/1, Scope/2
  Sin/1 -> Product18/1
  In4/1 -> Sum3/2
  Product18/1 -> Sum3/1
  Sum3/1 -> Square/1
  Sin3/1 -> Product19/1
  Product19/1 -> Sum8/1
  In3/1 -> Sum8/2
  Sum8/1 -> Square1/1
  Square/1 -> Sum9/1
  Square1/1 -> Sum9/2
  Sum9/1 -> Gain1/1
  In1/1 -> Product/2
  Transfer Fcn/1 -> Product/1
  Product/1 -> To Workspace/1, Product19/2, Product18/2
